simulink model "mbk"  (R2018a)
settings: Solver=ode4  StartTime=0.0  StopTime=50  FixedStep=0.01  RelTol=1e-3
InitFcn:
  | MBK
values from neighbouring files (symbols this model uses):
  b = 2    [MBK.m]
  k = 5    [MBK.m]
  m = 10    [MBK.m]
settings Model: Creator=Ali  LastModifiedBy=Ali

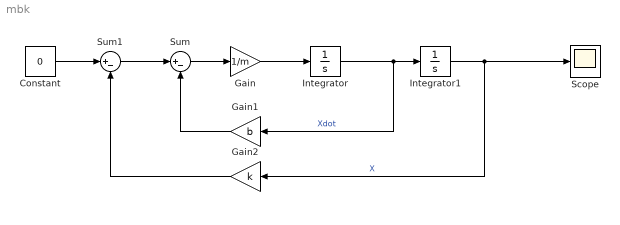
== system mbk ==
  Constant : Constant  Value=0
  Gain : Gain  Gain=1/m
  Gain1 : Gain  Gain=b
  Gain2 : Gain  Gain=k
  Integrator : Integrator  InitialCondition=1.5
  Integrator1 : Integrator  InitialCondition=3
  Scope : Scope
  Sum : Sum  Inputs=|+-
  Sum1 : Sum  Inputs=|+-
  wires:
  Integrator/1 -> Gain1/1, Integrator1/1  "Xdot"
  Integrator1/1 -> Gain2/1, Scope/1  "X"
  Gain/1 -> Integrator/1
  Sum/1 -> Gain/1
  Gain1/1 -> Sum/2
  Sum1/1 -> Sum/1
  Gain2/1 -> Sum1/2
  Constant/1 -> Sum1/1
